simulink model "regulator_parm_sim"  (R2024b)
settings: Solver=VariableStepAuto  StartTime=0.0  StopTime=2000  RelTol=1e-3
libraries: slpidlib x1
settings Model: Creator=michal  LastModifiedBy=michal

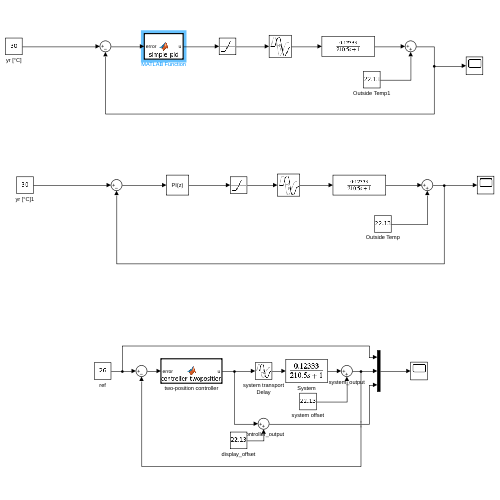
[thumbnail: Simulink's stored preview of the top-level diagram]
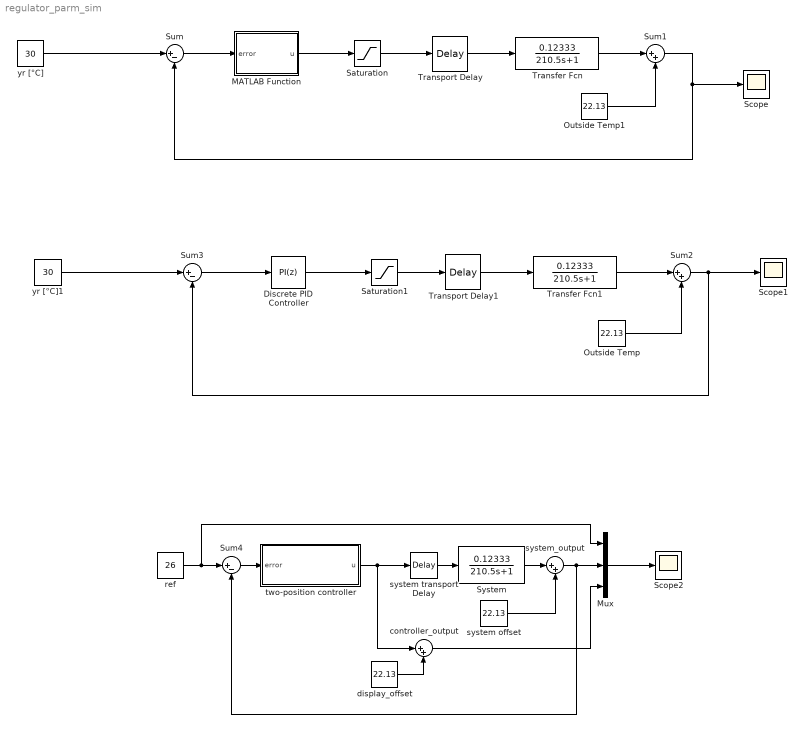
== system regulator_parm_sim ==
  Discrete PID Controller : slpidlib/PID Controller  Controller=PI  Form=Parallel  TimeDomain=Discrete-time  UseExternalTs=off  SampleTime=1  IntegratorMethod=Trapezoidal  FilterMethod=Forward Euler  ControllerParametersSource=internal  P=59.2041  I=0.34173  UseKiTs=off  D=0  UseExternalDerivativeSource=off  N=100  UseFilter=on  TunerSelectOption=Transfer Function Based (PID Tuner App)  InitialConditionSource=internal  InitialConditionForIntegrator=0  InitialConditionForFilter=0  DifferentiatorICPrevScaledInput=0  ExternalReset=none  TrackingMode=off  Kt=1  LimitOutput=off  SatLimitsSource=internal  UpperSaturationLimit=inf  LowerSaturationLimit=-inf  LinearizeAsGain=off  AntiWindupMode=none  Kb=1  LimitIntegrator=off  UpperIntegratorSaturationLimit=inf  LowerIntegratorSaturationLimit=-inf  POutMin=[]  POutMax=[]  IOutMin=[]  IOutMax=[]  DOutMin=[]  DOutMax=[]  NOutMin=[]  NOutMax=[]  SumOutMin=[]  SumOutMax=[]  SaturationOutMin=[]  SaturationOutMax=[]  PParamMin=[]  PParamMax=[]  IParamMin=[]  IParamMax=[]  DParamMin=[]  DParamMax=[]  NParamMin=[]  NParamMax=[]  KbParamMin=[]  KbParamMax=[]  KtParamMin=[]  KtParamMax=[]  KbOutMin=[]  KbOutMax=[]  KtOutMin=[]  KtOutMax=[]  IntegratorOutMin=[]  IntegratorOutMax=[]  FilterOutMin=[]  FilterOutMax=[]  SumI1OutMin=[]  SumI1OutMax=[]  SumI2OutMin=[]  SumI2OutMax=[]  SumI3OutMin=[]  SumI3OutMax=[]  SumI4OutMin=[]  SumI4OutMax=[]  SumDOutMin=[]  SumDOutMax=[]  DifferentiatorOutMin=[]  DifferentiatorOutMax=[]  FilterDiffOutCoefMin=[]  FilterDiffOutCoefMax=[]  ReciprocalOutMin=[]  ReciprocalOutMax=[]  SumDenOutMin=[]  SumDenOutMax=[]  SumNumOutMin=[]  SumNumOutMax=[]  DivideOutMin=[]  DivideOutMax=[]  UdiffTsProdOutMin=[]  UdiffTsProdOutMax=[]  NTsProdOutMin=[]  NTsProdOutMax=[]  UintegralTsProdOutMin=[]  UintegralTsProdOutMax=[]  UngainTsProdOutMin=[]  UngainTsProdOutMax=[]  ClampingZeroOutDataTypeStr=Inherit: Inherit via back propagation  ClampingZeroOutMin=[]  ClampingZeroOutMax=[]  FilterDenConstantOutDataTypeStr=Inherit: Inherit via back propagation  FilterDenConstantOutMin=[]  FilterDenConstantOutMax=[]  PCopyOutDataTypeStr=Inherit: Inherit via back propagation  PCopyOutMin=[]  PCopyOutMax=[]  NCopyOutDataTypeStr=Inherit: Inherit via back propagation  NCopyOutMin=[]  NCopyOutMax=[]  IntegratorContinuousStateAttributes=''  IntegratorStateMustResolveToSignalObject=off  IntegratorRTWStateStorageClass=Auto  FilterContinuousStateAttributes=''  FilterStateMustResolveToSignalObject=off  FilterRTWStateStorageClass=Auto  ParallelPVariant=InternalParameters  IdealPVariant=Disabled  IVariant=InternalParameters  DVariant=Disabled  IntegratorVariant=Discrete  SatVariant=Disabled  AWVariant=Passthrough  PCopyVariant=Disabled  TRVariant=Disabled  FdbkBlocksVariant=Forward  IdealPFdbkVariant=Disabled  SatFdbkVariant=Disabled  DerivativeFilterVariant=Disabled  NVariant=Disabled  NCopyVariant=Disabled_SignalSpec  FilterICVariant=Disabled  IntegratorICVariant=InternalICs  ExternalResetVariant=Disabled  TRSumVariant=Passthrough  SumFdbkVariant=Disabled  SumVariant=Sum_PI  TsampFilterVariant=InternalTs  TsampNgainVariant=Passthrough  TsampIntegralVariant=Disabled_SignalSpec  ExternalSaturationOutDataTypeStr=Inherit: Same as second input  DerivativeSourceVariant=Disabled  PreIntVariant=InternalPreInt
      settings: LibrarySourceBlock=simulink/Discrete/Discrete PID Controller
  MATLAB Function : MATLAB Function  TreatAsAtomicUnit=on
  Mux : Mux  Inputs=3
  Outside Temp : Constant  Value=22.13
  Outside Temp1 : Constant  Value=22.13
  Saturation : Saturate
  Saturation1 : Saturate
  Scope : Scope
  Scope1 : Scope
  Scope2 : Scope
  Sum : Sum  Inputs=|+-
  Sum1 : Sum  Inputs=|++
  Sum2 : Sum  Inputs=|++
  Sum3 : Sum  Inputs=|+-
  Sum4 : Sum  Inputs=|+-
  System : TransferFcn  Numerator=[0.12333]  Denominator=[210.5 1]
  Transfer Fcn : TransferFcn  Numerator=[0.12333]  Denominator=[210.5, 1]
  Transfer Fcn1 : TransferFcn  Numerator=[0.12333]  Denominator=[210.5, 1]
  Transport Delay : TransportDelay  DelayTime=10.9
  Transport Delay1 : TransportDelay  DelayTime=10.9
  controller_output : Sum  Inputs=|++
  display_offset : Constant  Value=22.13
  ref : Constant  Value=26
  system offset : Constant  Value=22.13
  system transport Delay : TransportDelay  DelayTime=10
  system_output : Sum  Inputs=|++
  two-position controller : MATLAB Function  TreatAsAtomicUnit=on
  yr [°C] : Constant  Value=30
  yr [°C]1 : Constant  Value=30
  wires:
  Discrete PID Controller/1 -> Saturation1/1
  Outside Temp/1 -> Sum2/2
  Sum2/1 -> Sum3/2, Scope1/1
  Sum3/1 -> Discrete PID Controller/1
  yr [°C]1/1 -> Sum3/1
  Saturation1/1 -> Transport Delay1/1
  Transport Delay1/1 -> Transfer Fcn1/1
  Transfer Fcn1/1 -> Sum2/1
  system_output/1 -> Mux/2, Sum4/2
  controller_output/1 -> Mux/3
  system transport Delay/1 -> System/1
  ref/1 -> Sum4/1, Mux/1
  System/1 -> system_output/1
  two-position controller/1(u) -> controller_output/1, system transport Delay/1
  system offset/1 -> system_output/2
  display_offset/1 -> controller_output/2
  Mux/1 -> Scope2/1
  Sum4/1 -> two-position controller/1(error)
  Transport Delay/1 -> Transfer Fcn/1
  Sum/1 -> MATLAB Function/1(error)
  MATLAB Function/1(u) -> Saturation/1
  Outside Temp1/1 -> Sum1/2
  Saturation/1 -> Transport Delay/1
  Transfer Fcn/1 -> Sum1/1
  yr [°C]/1 -> Sum/1
  Sum1/1 -> Sum/2, Scope/1

== matlab function regulator_parm_sim/two-position controller ==
  settings: updateMethod=DISCRETE
  data: u output; error input
function u = controller_twoposition(error)
%@author Dominik Łuczak

%Declare static value
persistent u_value;
if isempty(u_value)
    u_value = 0;
end

%Constant values
H = 0.5;
u_max = 1;
u_min = 0;

%Controller
if(error >= H/2) u_value=u_max; end
if(error < -H/2) u_value=u_min; end
    
u = u_value;

== matlab function regulator_parm_sim/MATLAB Function ==
  data: error input; u output
function u = simple_pid(error)

persistent previous_error;

if isempty(previous_error)
    previous_error = 0;
end

persistent previous_integral;

if isempty(previous_integral)
    previous_integral = 0;
end

dt = 1;
Kp = 59.2041;
Ki = 0.34173;
Kd = 0;
N = 100;

%Proportional part
P = Kp * error;

%Integral part
integral = previous_integral + (error + previous_error);
previous_integral = integral;
I = Ki * integral * (dt/2);


%Derivative Part
derivative = (error - previous_error)/dt;
previous_error = error;
D = Kd * derivative;

%Sum
u = P + I + D;
